simulink model "SatelliteSim"  (R2013a)
settings: Solver=ode45  StartTime=0.0  StopTime=1000  RelTol=1e-3
undefined symbols (not defined in the file or in its folder): drawSpacecraft, polar2cart
libraries: simulink x4
settings Model: Creator=Raj  LastModifiedBy=raj

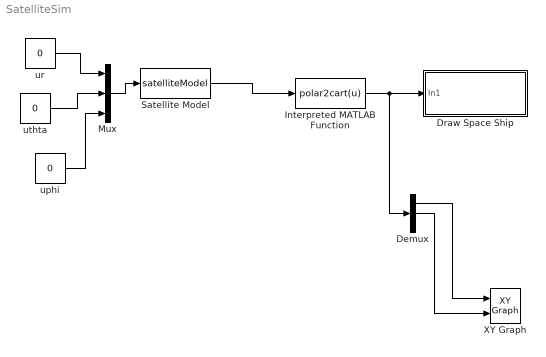
== system SatelliteSim ==
  Demux : Demux  Outputs=3
  Draw Space Ship : Subsystem
  Interpreted MATLAB Function : MATLABFcn  MATLABFcn=polar2cart(u)  OutputDimensions=3
  Mux : Mux  Inputs=3
  Satellite Model : S-Function  FunctionName=satelliteModel  Parameters=P  EnableBusSupport=off
  XY Graph : simulink/Sinks/XY Graph  xmin=- 7878  xmax=7878  ymin=- 7878  ymax=7878  st=-1
  uphi : Constant  Value=0
  ur : Constant  Value=0
  uthta : Constant  Value=0
  wires:
  ur/1 -> Mux/1
  uthta/1 -> Mux/2
  uphi/1 -> Mux/3
  Satellite Model/1 -> Interpreted MATLAB Function/1
  Mux/1 -> Satellite Model/1
  Interpreted MATLAB Function/1 -> Demux/1, Draw Space Ship/1(In1)
  Demux/1 -> XY Graph/1
  Demux/2 -> XY Graph/2

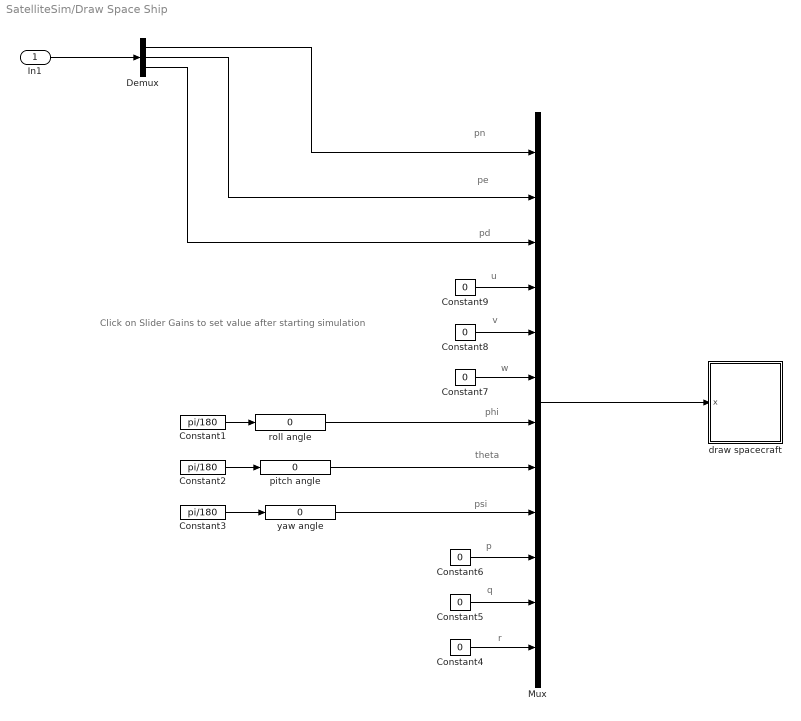
== system SatelliteSim/Draw Space Ship ==
  note: pn
  note: pe
  note: pd
  note: phi
  note: theta
  note: psi
  note: p
  note: q
  note: r
  note: u
  note: v
  note: w
  note: Click on Slider Gains to set value
      | after starting simulation
  In1 : Inport
  Constant1 : Constant  Value=pi/180
  Constant2 : Constant  Value=pi/180
  Constant3 : Constant  Value=pi/180
  Constant{4..9} (6 alike) : Constant  Value=0
  Demux : Demux  Outputs=3
  Mux : Mux  Inputs=12
  draw spacecraft : Subsystem
      mask init:
      | % define spacecraft points 
      | pts = [...
      | 	 1    1   0;... % point 1
      | 	 1   -1   0;... % point 2
      | 	-1   -1   0;... % point 3
      | 	-1    1   0;... % point 4
      |      1    1   0;... % point 1
      | 	 1    1  -2;... % point 5
      | 	 1   -1  -2;... % point 6
      | 	 1   -1   0;... % point 2
      | 	 1   -1  -2;... % point 6
      | 	-1   -1  -2;... % point 7
      | 	-1   -1   0;... % point 3
      | 	-1   -1  -2;... % point 7
      | 	-1    1  -2;... % point 8
      | 	-1    1   0;... % point 4
      | 	-1    1  -2;... % point 8
      | 	 1    1  -2;... % point 5
      | 	 1    1   0;... % point 1
      | 	 1.5  1.5 0;... % point 9
      | 	 1.5 -1.5 0;... % point 10
      | 	 1   -1   0;... % point 2
      | 	 1.5 -1.5 0;... % point 10
      | 	-1.5 -1.5 0;... % point 11
      | 	-1   -1   0;... % point 3
      | 	-1.5 -1.5 0;... % point 11
      | 	-1.5  1.5 0;... % point 12
      | 	-1    1   0;... % point 4
      | 	-1.5  1.5 0;... % point 12
      | 	 1.5  1.5 0;... % point 9
      |   ]';
      mask Display: image(imread('tv.jpg'))
  pitch angle : simulink/Math Operations/Slider Gain  low=-180  gain=0  high=180
  roll angle : simulink/Math Operations/Slider Gain  low=-180  gain=0  high=180
  "yaw angle " : simulink/Math Operations/Slider Gain  low=-180  gain=0  high=180
  wires:
  Mux/1 -> draw spacecraft/1(x)
  roll angle/1 -> Mux/7
  Constant1/1 -> roll angle/1
  pitch angle/1 -> Mux/8
  Constant2/1 -> pitch angle/1
  "yaw angle "/1 -> Mux/9
  Constant3/1 -> "yaw angle "/1
  Constant4/1 -> Mux/12
  Constant5/1 -> Mux/11
  Constant6/1 -> Mux/10
  Constant7/1 -> Mux/6
  Constant8/1 -> Mux/5
  Constant9/1 -> Mux/4
  Demux/1 -> Mux/1
  Demux/2 -> Mux/2
  Demux/3 -> Mux/3
  In1/1 -> Demux/1

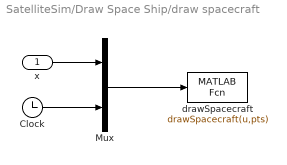
== system SatelliteSim/Draw Space Ship/draw spacecraft ==
  x : Inport
  Clock : Clock
  Mux : Mux  Inputs=2
  drawSpacecraft : MATLABFcn  MATLABFcn=drawSpacecraft(u,pts)  OutputDimensions=0  SampleTime=0.1
  wires:
  Mux/1 -> drawSpacecraft/1
  x/1 -> Mux/1
  Clock/1 -> Mux/2
